simulink library "CTRL_SPECCTRL_FB_COND"  (R2024b)
settings: Solver=VariableStepAuto  StartTime=0.0  StopTime=10.0  RelTol=1e-3
settings Model: Creator=blatak  LastModifiedBy=blatak

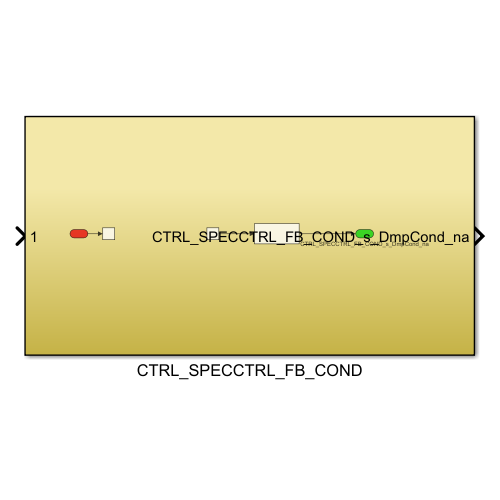
[thumbnail: Simulink's stored preview of the top-level diagram]
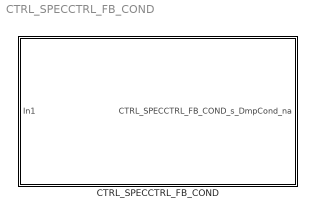
== system CTRL_SPECCTRL_FB_COND ==
  CTRL_SPECCTRL_FB_COND : Subsystem

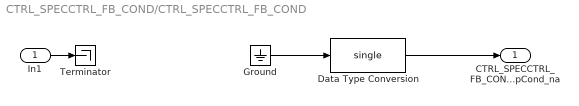
== system CTRL_SPECCTRL_FB_COND/CTRL_SPECCTRL_FB_COND ==
  In1 : Inport
  Data Type Conversion : DataTypeConversion  OutDataTypeStr=single  SaturateOnIntegerOverflow=off  RndMeth=Floor
  Ground : Ground
  Terminator : Terminator
  CTRL_SPECCTRL_FB_COND_s_DmpCond_na : Outport
  wires:
  In1/1 -> Terminator/1
  Ground/1 -> Data Type Conversion/1
  Data Type Conversion/1 -> CTRL_SPECCTRL_FB_COND_s_DmpCond_na/1
